simulink model "leg"  (R2022b)
settings: Solver=ode23  StartTime=0.0  StopTime=10  MaxStep=0.1  RelTol=1e-3
model workspace: external: MATLAB File D:\Avaritia\Projects\MATLAB\leg\leg_DataFile.m (data not in the file)
undefined symbols (not defined in the file or in its folder): smiData, X, Y, Z
libraries: sm_lib x46, nesl_utility x5, simulink_extras x4
(part 2 of 2)

== matlab function leg/joint values ==
  data: theta1 output; theta2 output; t input
function [theta1, theta2] = joint(t)

    tf = 1;

    joint1_array = [34 56 60 66 72 81 79 76 71 56];
    
    joint2_array = [106 98 112 117 132 115 85 66 60 80];
          
    if t==0 || t<=1 
        theta1_0 = joint1_array(1);
        theta1_f = joint1_array(2);
        a0 = theta1_0;
        a1 = 0;
        a2 = (3*(theta1_f - theta1_0))/tf^2;
        a3 = (-2*(theta1_f - theta1_0))/tf^3;
        theta1 = a0 + a1*t + a2*t^2 + a3*t^3;
        theta2_0 = joint2_array(1);
        theta2_f = joint2_array(2);
        b0 = theta2_0;
        b1 = 0;
        b2 = 3*(theta2_f - theta2_0)/tf^2;
        b3 = -2*(theta2_f - theta2_0)/tf^3;
        theta2 = b0 + b1*t + b2*t^2 + b3*t^3;

    elseif t>=1 && t<=2
        t1=t-1;
        theta1_0 = joint1_array(2);
        theta1_f = joint1_array(3);
        a0 = theta1_0;
        a1 = 0;
        a2 = (3*(theta1_f - theta1_0))/tf^2;
        a3 = (-2*(theta1_f - theta1_0))/tf^3;
        theta1 = a0 + a1*t1 + a2*t1^2 + a3*t1^3;
        theta2_0 = joint2_array(2);
        theta2_f = joint2_array(3);
        b0 = theta2_0;
        b1 = 0;
        b2 = 3*(theta2_f - theta2_0)/tf^2;
        b3 = -2*(theta2_f - theta2_0)/tf^3;
        theta2 = b0 + b1*t1 + b2*t1^2 + b3*t1^3;

    elseif t>=2 && t<=3
        t1=t-2;
        theta1_0 = joint1_array(3);
        theta1_f = joint1_array(4);
        a0 = theta1_0;
        a1 = 0;
        a2 = (3*(theta1_f - theta1_0))/tf^2;
        a3 = (-2*(theta1_f - theta1_0))/tf^3;
        theta1 = a0 + a1*t1 + a2*t1^2 + a3*t1^3;
        theta2_0 = joint2_array(3);
        theta2_f = joint2_array(4);
        b0 = theta2_0;
        b1 = 0;
        b2 = 3*(theta2_f - theta2_0)/tf^2;
        b3 = -2*(theta2_f - theta2_0)/tf^3;
        theta2 = b0 + b1*t1 + b2*t1^2 + b3*t1^3;

    elseif t>=3 && t<=4
        t1=t-3;
        theta1_0 = joint1_array(4);
        theta1_f = joint1_array(5);
        a0 = theta1_0;
        a1 = 0;
        a2 = (3*(theta1_f - theta1_0))/tf^2;
        a3 = (-2*(theta1_f - theta1_0))/tf^3;
        theta1 = a0 + a1*t1 + a2*t1^2 + a3*t1^3;
        theta2_0 = joint2_array(4);
        theta2_f = joint2_array(5);
        b0 = theta2_0;
        b1 = 0;
        b2 = 3*(theta2_f - theta2_0)/tf^2;
        b3 = -2*(theta2_f - theta2_0)/tf^3;
        theta2 = b0 + b1*t1 + b2*t1^2 + b3*t1^3;

    elseif t>=4 && t<=5
        t1=t-4;
        theta1_0 = joint1_array(5);
        theta1_f = joint1_array(6);
        a0 = theta1_0;
        a1 = 0;
        a2 = (3*(theta1_f - theta1_0))/tf^2;
        a3 = (-2*(theta1_f - theta1_0))/tf^3;
        theta1 = a0 + a1*t1 + a2*t1^2 + a3*t1^3;
        theta2_0 = joint2_array(5);
        theta2_f = joint2_array(6);
        b0 = theta2_0;
        b1 = 0;
        b2 = 3*(theta2_f - theta2_0)/tf^2;
        b3 = -2*(theta2_f - theta2_0)/tf^3;
        theta2 = b0 + b1*t1 + b2*t1^2 + b3*t1^3;

    elseif t>=5 && t<=6
        t1=t-5;
        theta1_0 = joint1_array(6);
        theta1_f = joint1_array(7);
        a0 = theta1_0;
        a1 = 0;
        a2 = (3*(theta1_f - theta1_0))/tf^2;
        a3 = (-2*(theta1_f - theta1_0))/tf^3;
        theta1 = a0 + a1*t1 + a2*t1^2 + a3*t1^3;
        theta2_0 = joint2_array(6);
        theta2_f = joint2_array(7);
        b0 = theta2_0;
        b1 = 0;
        b2 = 3*(theta2_f - theta2_0)/tf^2;
        b3 = -2*(theta2_f - theta2_0)/tf^3;
        theta2 = b0 + b1*t1 + b2*t1^2 + b3*t1^3;

    elseif t>=6 && t<=7
        t1=t-6;
        theta1_0 = joint1_array(7);
        theta1_f = joint1_array(8);
        a0 = theta1_0;
        a1 = 0;
        a2 = (3*(theta1_f - theta1_0))/tf^2;
        a3 = (-2*(theta1_f - theta1_0))/tf^3;
        theta1 = a0 + a1*t1 + a2*t1^2 + a3*t1^3;
        theta2_0 = joint2_array(7);
        theta2_f = joint2_array(8);
        b0 = theta2_0;
        b1 = 0;
        b2 = 3*(theta2_f - theta2_0)/tf^2;
        b3 = -2*(theta2_f - theta2_0)/tf^3;
        theta2 = b0 + b1*t1 + b2*t1^2 + b3*t1^3;

    elseif t>=7 && t<=8
        t1=t-7;
        theta1_0 = joint1_array(8);
        theta1_f = joint1_array(9);
        a0 = theta1_0;
        a1 = 0;
        a2 = (3*(theta1_f - theta1_0))/tf^2;
        a3 = (-2*(theta1_f - theta1_0))/tf^3;
        theta1 = a0 + a1*t1 + a2*t1^2 + a3*t1^3;
        theta2_0 = joint2_array(8);
        theta2_f = joint2_array(9);
        b0 = theta2_0;
        b1 = 0;
        b2 = 3*(theta2_f - theta2_0)/tf^2;
        b3 = -2*(theta2_f - theta2_0)/tf^3;
        theta2 = b0 + b1*t1 + b2*t1^2 + b3*t1^3;

    elseif t>=8 && t<=9
        t1=t-8;
        theta1_0 = joint1_array(9);
        theta1_f = joint1_array(10);
        a0 = theta1_0;
        a1 = 0;
        a2 = (3*(theta1_f - theta1_0))/tf^2;
        a3 = (-2*(theta1_f - theta1_0))/tf^3;
        theta1 = a0 + a1*t1 + a2*t1^2 + a3*t1^3;
        theta2_0 = joint2_array(9);
        theta2_f = joint2_array(10);
        b0 = theta2_0;
        b1 = 0;
        b2 = 3*(theta2_f - theta2_0)/tf^2;
        b3 = -2*(theta2_f - theta2_0)/tf^3;
        theta2 = b0 + b1*t1 + b2*t1^2 + b3*t1^3;

    elseif t>=9 && t<=10
        t1=t-9;
        theta1_0 = joint1_array(10);
        theta1_f = joint1_array(1);
        a0 = theta1_0;
        a1 = 0;
        a2 = (3*(theta1_f - theta1_0))/tf^2;
        a3 = (-2*(theta1_f - theta1_0))/tf^3;
        theta1 = a0 + a1*t1 + a2*t1^2 + a3*t1^3;
        theta2_0 = joint2_array(10);
        theta2_f = joint2_array(1);
        b0 = theta2_0;
        b1 = 0;
        b2 = 3*(theta2_f - theta2_0)/tf^2;
        b3 = -2*(theta2_f - theta2_0)/tf^3;
        theta2 = b0 + b1*t1 + b2*t1^2 + b3*t1^3;

    else
        theta1=0;
        theta2=0;
        
    end
